simulink model "switched_simstate_realization"  (R2020a)
settings: Solver=FixedStepAuto  StartTime=22  StopTime=42  FixedStep=dt  RelTol=1e-3
values from neighbouring files (symbols this model uses):
  dt = 0.001    [param_init.m]    (also in sim_switched.m = options.dt)
undefined symbols (not defined in the file or in its folder): Ap, Bp, Cp, Dp
libraries: simulink x1
settings Model: Creator=kekatos  LastModifiedBy=kekatos
settings DataIOCC: FinalStateName=SimState  InitialState=SimState_previous  LoadInitialState=on  SaveFinalState=on  DSMLogging=off  ReturnWorkspaceOutputs=off

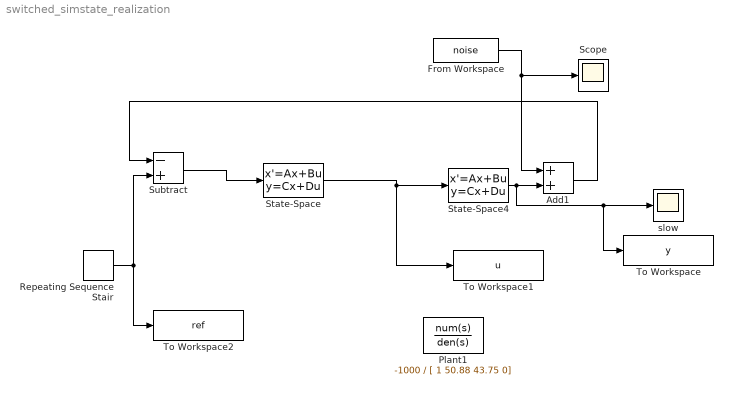
== system switched_simstate_realization ==
  Add1 : Sum
  From Workspace : FromWorkspace  VariableName=noise
  Plant1 : TransferFcn  Numerator=-1000  Denominator=[ 1 50.88 43.75 0]
  Repeating Sequence Stair : simulink/Sources/Repeating Sequence Stair  OutValues=[1 1 1 1 1 0 0 0 0 0].'  tsamp=2  OutMin=[]  OutMax=[]  OutDataTypeStr=double  OutputDataTypeScalingMode=double  OutDataType=fixdt(0,8)  ConRadixGroup=Best Precision: Vector-wise  OutScaling=2^-12
  Scope : Scope
  State-Space : StateSpace  A=[-63.28 -23.49 -8.735 ; 32 0 0;0 16 0]  B=[ 4 0 0]'  C=[-1.673 -2.665 -0.1544]  D=0  InitialCondition=[-0.0010 , -0.0000,0.0000]
  State-Space4 : StateSpace  A=Ap  B=Bp  C=Cp  D=Dp  InitialCondition=0
  Subtract : Sum  Inputs=-+
  To Workspace : ToWorkspace  VariableName=y  SaveFormat=Structure With Time  SampleTime=dt
  To Workspace1 : ToWorkspace  VariableName=u  SaveFormat=Structure With Time  SampleTime=dt
  To Workspace2 : ToWorkspace  VariableName=ref  SaveFormat=Structure With Time  SampleTime=dt
  slow : Scope
  wires:
  State-Space4/1 -> To Workspace/1, slow/1, Add1/2
  Subtract/1 -> State-Space/1
  State-Space/1 -> State-Space4/1, To Workspace1/1
  Repeating Sequence Stair/1 -> To Workspace2/1, Subtract/2
  Add1/1 -> Subtract/1
  From Workspace/1 -> Scope/1, Add1/1
